simulink model "lookupTableDynamic_TestGen23"  (R2017b)
settings: Solver=FixedStepDiscrete  StartTime=0.0  StopTime=10.0  RelTol=1e-3
libraries: simulink x1
settings Model: Creator=ktrinh  LastModifiedBy=ktrinh
settings DebuggingCC: ParameterOverflowMsg=none

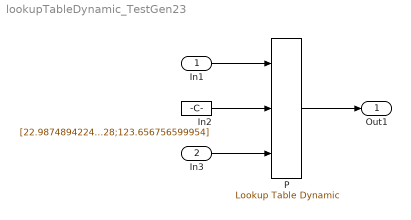
== system lookupTableDynamic_TestGen23 ==
  In1 : Inport  OutMin=20.9875  OutMax=126  OutDataTypeStr=int32  PortDimensions=[2,3]
  In3 : Inport  Port=2  PortDimensions=5
  In2 : Constant  Value=[22.9874894224613;32.0928290672108;59.1893145796931;59.3309797134328;123.656756599954]  OutDataTypeStr=int32
  P : simulink/Lookup Tables/Lookup Table Dynamic  LookUpMeth=Use Input Nearest  OutDataType=fixdt('int16')  OutScaling=[]  OutputDataTypeScalingMode=Specify via dialog  OutDataTypeStr=int16  DoSatur=on
      settings: SourceProductName=Simulink
  Out1 : Outport
  wires:
  In1/1 -> P/1
  In2/1 -> P/2
  In3/1 -> P/3
  P/1 -> Out1/1
